simulink model "position_control"  (R2024b)
settings: Solver=FixedStepAuto  StartTime=0.0  StopTime=t_end  FixedStep=dt  RelTol=1e-3
undefined symbols (not defined in the file or in its folder): kp, p_init, p_r
settings Model: Creator=yamauchi  LastModifiedBy=yamauchi

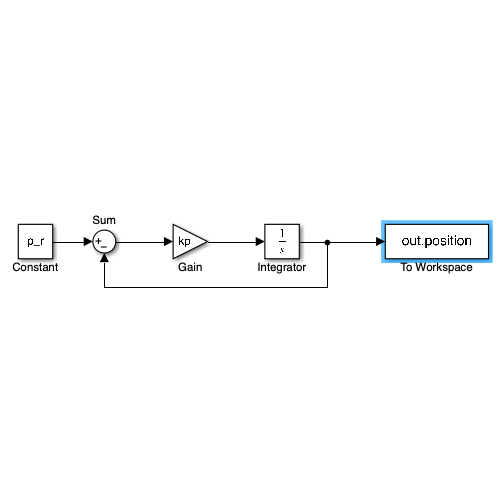
[thumbnail: Simulink's stored preview of the top-level diagram]
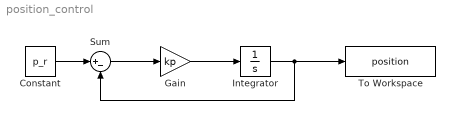
== system position_control ==
  Constant : Constant  Value=p_r
  Gain : Gain  Gain=kp
  Integrator : Integrator  InitialCondition=p_init
  Sum : Sum  Inputs=|+-
  To Workspace : ToWorkspace  VariableName=position  SampleTime=-1
      settings: Save2DSignal=2-D array (concatenate along first dimension)
  wires:
  Gain/1 -> Integrator/1
  Constant/1 -> Sum/1
  Sum/1 -> Gain/1
  Integrator/1 -> To Workspace/1, Sum/2
